simulink model "Half_car_model_susp_bump_tyre"  (R2025b)
settings: Solver=VariableStepAuto  StartTime=0.0  StopTime=15  RelTol=1e-3
values from neighbouring files (symbols this model uses):
  A_N = double(vpa(subs(A_0, symbol_vars , numeric_vals), 6))    [half_car_active_suspensions_bump.m]
  B1_N = double(vpa(subs(B1_0, symbol_vars , numeric_vals), 6))    [half_car_active_suspensions_bump.m]
  B2_N = double(vpa(subs(B2_0, symbol_vars , numeric_vals), 6))    [half_car_active_suspensions_bump.m]
  bump_t_dist = (df+dr)/1    (= 3)    [half_car_active_suspensions_bump.m]
  C_N = double(vpa(subs(C_0, symbol_vars , numeric_vals), 6))    [half_car_active_suspensions_bump.m]
  CE_N = double(vpa(subs(CE_0, symbol_vars , numeric_vals), 6))    [half_car_active_suspensions_bump.m]
  D1_N = double(vpa(subs(D1_0, symbol_vars , numeric_vals), 6))    [half_car_active_suspensions_bump.m]
  D2_N = double(vpa(subs(D2_0, symbol_vars , numeric_vals), 6))    [half_car_active_suspensions_bump.m]
  DE2_N = double(vpa(subs(DE2_0, symbol_vars , numeric_vals), 6))    [half_car_active_suspensions_bump.m]
  Delta0 = -(m)*g/(2*k)    (= -0.17658)    [half_car_active_suspensions_bump.m]
  Delta0_W = -(m+mwf*2)*g/(2*ktf)    (= -0.0230535)    [half_car_active_suspensions_bump.m]
  Ko = place(A_N', C_N', poles_obs)'    [half_car_active_suspensions_bump.m]
  Ks = [Ks_c, zeros(2, 4)]    [half_car_active_suspensions_bump.m]
  Ks_obs = lqr(A_stabile, B1_N, Q, R)    [half_car_active_suspensions_bump.m]
  par_numeric = [ m, k, beta, ell0, g, df, dr, J, mwf, mwr, ktf, ktr ]    [half_car_active_suspensions_bump.m]
  u0 = [0; 0]    [half_car_active_suspensions_bump.m]
  x0 = [  Delta0 + Delta0_W ... (first row only)    [half_car_active_suspensions_bump.m]
  x0_lin = [ ... (first row only)    [half_car_active_suspensions_bump.m]
libraries: simulink x1
settings Model: LastModifiedBy=alex2

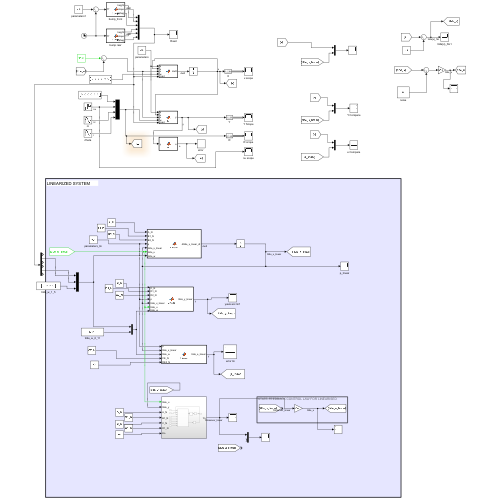
[thumbnail: Simulink's stored preview of the top-level diagram]
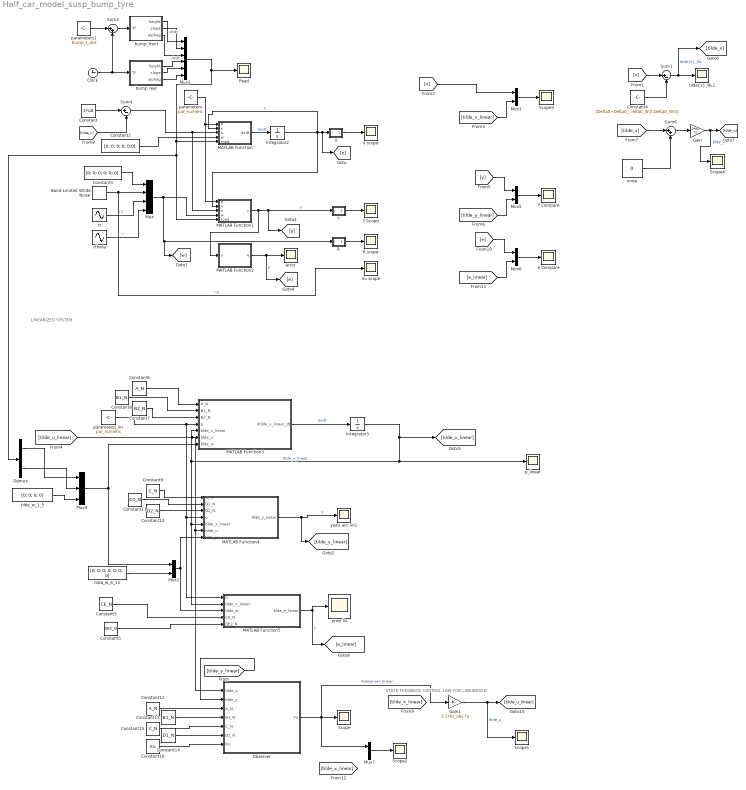
== system Half_car_model_susp_bump_tyre ==
  note: STATE-FEEDBACK CONTROL LAW FOR LINEARISED
  note: LINEARIZED SYSTEM
  " error lin" : Scope
      settings: ActiveDisplayYMinimum=-1  ActiveDisplayYMaximum=1  DataLoggingVariableName=ScopeData8
  Band-Limited White Noise : simulink/Sources/Band-Limited White Noise  Cov="1*[0.00001*1e-2; 0.00001*1e-2;  0.00001*1e-2; 0.00001*1e-2; 0.00001*1e-2]"  Ts=1e-2  seed=[23341; 31826; 11111; 81818; 00001]
  Clock : Clock
  Constant : Constant  Value=1*u0
  Constant1 : Constant  Value=[0; 0; 0; 0; 0; 0]
  Constant10 : Constant  Value=D2_N
  Constant11 : Constant  Value=D1_N
  Constant12 : Constant  Value=A_N
  Constant13 : Constant  Value=B1_N
  Constant14 : Constant  Value=D1_N
  Constant15 : Constant  Value=C_N
  Constant16 : Constant  Value=Ko
  Constant2 : Constant  Value=[0; 0; 0; 0; 0;0]
  Constant3 : Constant  Value=CE_N
  Constant4 : Constant  Value=[Delta0+Delta0_W;0;0;0;Delta0_W;0;Delta0_W;0]
  Constant5 : Constant  Value=DE2_N
  Constant6 : Constant  Value=A_N
  Constant7 : Constant  Value=B2_N
  Constant8 : Constant  Value=B1_N
  Constant9 : Constant  Value=C_N
  Demux : Demux  Outputs=6
  Gain : Gain  Gain=0*Ks  Multiplication=Matrix(K*u)
  Gain1 : Gain  Gain=3.5*Ks_obs  Multiplication=Matrix(K*u)
  Integrator2 : Integrator  InitialCondition=x0
  Integrator3 : Integrator  InitialCondition=x0_lin
  MATLAB Function : MATLAB Function  TreatAsAtomicUnit=on
  MATLAB Function1 : MATLAB Function  TreatAsAtomicUnit=on
  MATLAB Function2 : MATLAB Function  TreatAsAtomicUnit=on
  MATLAB Function3 : MATLAB Function  TreatAsAtomicUnit=on
  MATLAB Function4 : MATLAB Function  TreatAsAtomicUnit=on
  MATLAB Function5 : MATLAB Function  TreatAsAtomicUnit=on
  Mux : Mux
  Mux{1..2,5..7} (5 alike) : Mux  Inputs=2
  Mux3 : Mux  Inputs=6
  Mux4 : Mux  Inputs=3
  Observer : Subsystem
  R : Subsystem
  R scope : Scope
      settings: ActiveDisplayYMinimum=-1  ActiveDisplayYMaximum=1  DataLoggingVariableName=ScopeData5
  Road : Scope
      settings: ActiveDisplayYMinimum=-0.19634954084936207  ActiveDisplayYMaximum=0.19634954084936207
  Scope{,1..4} (5 alike) : Scope
      Scope settings: ActiveDisplayYMinimum=-1  ActiveDisplayYMaximum=1  DataLoggingVariableName=ScopeData13
      Scope1 settings: ActiveDisplayYMinimum=-1  ActiveDisplayYMaximum=1  DataLoggingVariableName=ScopeData14
      Scope2 settings: ActiveDisplayYMinimum=-1.3124834996188637  ActiveDisplayYMaximum=1.3703591925048633  DataLoggingVariableName=ScopeData15
      Scope3 settings: ActiveDisplayYMinimum=-0.26211296691734631  ActiveDisplayYMaximum=0.090134709396633
      Scope4 settings: ActiveDisplayYMinimum=-1  ActiveDisplayYMaximum=1  DataLoggingVariableName=ScopeData16
  Sum1 : Sum  Inputs=|+-
  Sum2 : Sum  Inputs=|++
  Sum4 : Sum  Inputs=|+-
  Sum6 : Sum  Inputs=|++
  X : Subsystem
  Y : Subsystem
  Y Compare : Scope
      settings: ActiveDisplayYMinimum=-9.06978679583773  ActiveDisplayYMaximum=22.15478865739642  DataLoggingVariableName=ScopeData11
  Y Scope : Scope
      settings: ActiveDisplayYMinimum=-1  ActiveDisplayYMaximum=1  DataLoggingVariableName=ScopeData3
  bump rear : MATLAB Function  TreatAsAtomicUnit=on
  bump_front : MATLAB Function  TreatAsAtomicUnit=on
  e Compare : Scope
      settings: ActiveDisplayYMinimum=-0.3208309292462625  ActiveDisplayYMaximum=0.34771769859425983  DataLoggingVariableName=ScopeData12
  "error " : Scope
      settings: ActiveDisplayYMinimum=-1  ActiveDisplayYMaximum=1  DataLoggingVariableName=ScopeData6
  noise : Constant  Value=0
  nu scope : Scope
      settings: DataLoggingVariableName=ScopeData7
  p_linear : Scope
      settings: ActiveDisplayYMinimum=-0.03749851288711617  ActiveDisplayYMaximum=0.066646245320476569  DataLoggingVariableName=ScopeData9
  parameters : Constant  Value=par_numeric  VectorParams1D=off
  parameters1 : Constant  Value=bump_t_dist  VectorParams1D=off
  parameters_lin : Constant  Value=par_numeric
  rtheta : Sin  Amplitude=0  Frequency=0  SampleTime=0
  rz : Sin  Amplitude=0  Frequency=0  SampleTime=0
  tilde_w_1_5 : Constant  Value=[0; 0; 0; 0]
  tilde_w_6_11 : Constant  Value=[0; 0; 0; 0; 0; 0; 0]
  "tilde{x}_NL1" : Scope
      settings: ActiveDisplayYMinimum=-4.93552  ActiveDisplayYMaximum=2.55492  DataLoggingVariableName=ScopeData4
  x scope : Scope
      settings: ActiveDisplayYMinimum=-0.66741875872169254  ActiveDisplayYMaximum=0.73384060742897  DataLoggingVariableName=ScopeData2
  yaxis acc lin1 : Scope
      settings: ActiveDisplayYMinimum=-1  ActiveDisplayYMaximum=1  DataLoggingVariableName=ScopeData10
  wires:
  Clock/1 -> Sum2/2, bump rear/1(Tf)
  bump_front/2(slope) -> Mux3/2
  Sum2/1 -> bump_front/1(Tf)
  parameters1/1 -> Sum2/1
  Mux3/1 -> Road/1, MATLAB Function/5(road), Demux/1, MATLAB Function1/5(road)
  bump_front/1(height) -> Mux3/1  "dxdt"
  Constant/1 -> Sum4/1
  Sum4/1 -> MATLAB Function1/3(u), MATLAB Function/3(u)
  Constant2/1 -> MATLAB Function/4(w)
  MATLAB Function/1(dxdt) -> Integrator2/1  "dxdt"
  MATLAB Function1/1(y) -> Y/1(i), [y], MATLAB Function2/1(y)  "y"
  Constant1/1 -> Mux/1
  rtheta/1 -> Mux/4  "r"
  parameters/1 -> MATLAB Function1/1(p), MATLAB Function/1(p)
  Band-Limited White Noise/1 -> nu scope/1, Mux/2  "nu"
  rz/1 -> Mux/3  "rz"
  Mux/1 -> [w], R/1(i), MATLAB Function1/4(w)
  MATLAB Function2/1(e) -> [e], "error "/1  "e"
  Sum6/1 -> Gain/1
  [tilde_x] -> Sum6/1
  [x] -> Sum1/1
  Constant4/1 -> Sum1/2
  Sum1/1 -> [tilde_x], "tilde{x}_NL1"/1  "tilde{x}_NL"
  noise/1 -> Sum6/2
  [tilde_x_linear] -> Mux1/2
  Gain/1 -> Scope4/1, [tilde_u]  "tilde_u"
  Mux1/1 -> Scope3/1
  [tilde_u] -> Sum4/2
  Integrator2/1 -> [x], X/1(i), MATLAB Function1/2(x), MATLAB Function/2(x)  "x"
  X/1(o) -> x scope/1
  Y/1(o) -> Y Scope/1
  R/1(o) -> R scope/1
  tilde_w_6_11/1 -> Mux2/2
  parameters_lin/1 -> MATLAB Function3/4(p), MATLAB Function5/1(p), MATLAB Function4/4(p)
  [tilde_u_linear] -> Observer/1(tilde_u), MATLAB Function4/6(tilde_u), MATLAB Function3/6(tilde_u)
  Gain1/1 -> Scope1/1, [tilde_u_linear]  "tilde_u"
  MATLAB Function4/1(tilde_y_linear) -> [tilde_y_linear], yaxis acc lin1/1  "y"
  Mux2/1 -> MATLAB Function4/7(tilde_w), MATLAB Function5/3(tilde_w)
  MATLAB Function5/1(tilde_e_linear) -> " error lin"/1, [e_linear]  "y"
  Constant3/1 -> MATLAB Function5/4(CE_N)
  Constant5/1 -> MATLAB Function5/5(DE2_N)
  Constant7/1 -> MATLAB Function3/3(B2_N)
  Constant6/1 -> MATLAB Function3/1(A_N)
  Constant8/1 -> MATLAB Function3/2(B1_N)
  Constant10/1 -> MATLAB Function4/3(D2_N)
  Constant11/1 -> MATLAB Function4/2(D1_N)
  Constant9/1 -> MATLAB Function4/1(C_N)
  Mux4/1 -> MATLAB Function3/7(tilde_w), Mux2/1
  tilde_w_1_5/1 -> Mux4/3
  Demux/2 -> Mux4/1
  bump_front/3(alphag) -> Mux3/3
  bump rear/1(height) -> Mux3/4  "dxdt"
  bump rear/2(slope) -> Mux3/5
  bump rear/3(alphag) -> Mux3/6
  Demux/5 -> Mux4/2
  MATLAB Function3/1(dtilde_x_linear_dt) -> Integrator3/1  "dxdt"
  Integrator3/1 -> p_linear/1, MATLAB Function3/5(tilde_x_linear), MATLAB Function5/2(tilde_x_linear), MATLAB Function4/5(tilde_x_linear), [tilde_x_linear]  "tilde_x_linear"
  [y] -> Mux5/1
  Mux5/1 -> Y Compare/1
  [tilde_y_linear] -> Mux5/2
  Mux6/1 -> e Compare/1
  [e] -> Mux6/1
  [e_linear] -> Mux6/2
  [tilde_y_linear] -> Observer/2(tilde_y)
  Observer/1(Yo) -> Mux7/1, Gain1/1, Scope/1  "Yobserver_linear"
  Constant16/1 -> Observer/7(Ko)
  Constant14/1 -> Observer/6(D1_N)
  Constant15/1 -> Observer/5(C_N)
  Constant13/1 -> Observer/4(B1_N)
  Constant12/1 -> Observer/3(A_N)
  Mux7/1 -> Scope2/1
  [x] -> Mux1/1

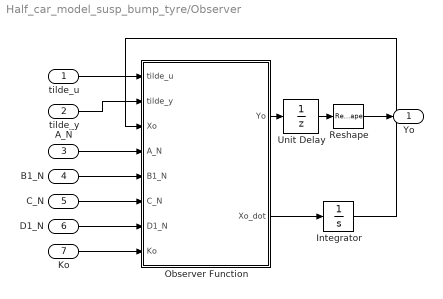
== system Half_car_model_susp_bump_tyre/Observer ==
  tilde_u : Inport
  tilde_y : Inport  Port=2
  A_N : Inport  Port=3
  B1_N : Inport  Port=4
  C_N : Inport  Port=5
  D1_N : Inport  Port=6
  Ko : Inport  Port=7
  Integrator : Integrator  InitialCondition=x0_lin
  Observer Function : MATLAB Function  TreatAsAtomicUnit=on
  Reshape : Reshape  OutputDimensionality=Customize  OutputDimensions=[12]
  Unit Delay : UnitDelay  SampleTime=0.01  HasFrameUpgradeWarning=on
  Yo : Outport
  wires:
  Observer Function/2(Xo_dot) -> Integrator/1
  Integrator/1 -> Observer Function/3(Xo)
  tilde_u/1 -> Observer Function/1(tilde_u)
  tilde_y/1 -> Observer Function/2(tilde_y)
  A_N/1 -> Observer Function/4(A_N)
  B1_N/1 -> Observer Function/5(B1_N)
  C_N/1 -> Observer Function/6(C_N)
  D1_N/1 -> Observer Function/7(D1_N)
  Ko/1 -> Observer Function/8(Ko)
  Reshape/1 -> Yo/1
  Observer Function/1(Yo) -> Unit Delay/1
  Unit Delay/1 -> Reshape/1

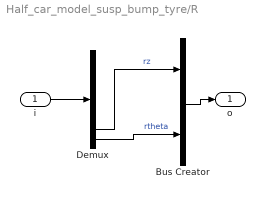
== system Half_car_model_susp_bump_tyre/R ==
  i : Inport
  Bus Creator : BusCreator  Inputs=2
  Demux : Demux  Outputs=9
  o : Outport
  wires:
  i/1 -> Demux/1
  Bus Creator/1 -> o/1
  Demux/9 -> Bus Creator/2  "rtheta"
  Demux/8 -> Bus Creator/1  "rz"

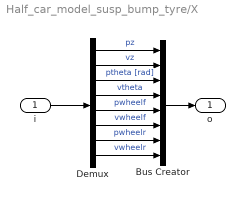
== system Half_car_model_susp_bump_tyre/X ==
  i : Inport
  Bus Creator : BusCreator  Inputs=8
  Demux : Demux  Outputs=8
  o : Outport
  wires:
  Demux/8 -> Bus Creator/8  "vwheelr"
  Demux/4 -> Bus Creator/4  "vtheta"
  Demux/1 -> Bus Creator/1  "pz"
  Demux/2 -> Bus Creator/2  "vz"
  Demux/5 -> Bus Creator/5  "pwheelf"
  Demux/3 -> Bus Creator/3  "ptheta [rad]"
  Demux/7 -> Bus Creator/7  "pwheelr"
  Demux/6 -> Bus Creator/6  "vwheelf"
  i/1 -> Demux/1
  Bus Creator/1 -> o/1

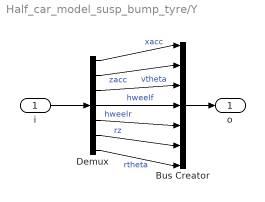
== system Half_car_model_susp_bump_tyre/Y ==
  i : Inport
  Bus Creator : BusCreator  Inputs=7
  Demux : Demux  Outputs=7
  o : Outport
  wires:
  Demux/4 -> Bus Creator/4  "hweelf"
  Demux/1 -> Bus Creator/1  "xacc"
  Demux/2 -> Bus Creator/2  "zacc"
  Demux/3 -> Bus Creator/3  "vtheta"
  i/1 -> Demux/1
  Bus Creator/1 -> o/1
  Demux/7 -> Bus Creator/7  "rtheta"
  Demux/6 -> Bus Creator/6  "rz"
  Demux/5 -> Bus Creator/5  "hweelr"

== matlab function Half_car_model_susp_bump_tyre/MATLAB Function1 ==
  data: p input; x input; u input; y output; w input; road input
function y = h(p,x, u, w, road)

%% parameters
m = p(1);      % [kg] mass
k = p(2);    % [N/m] spring stiffness
beta = p(3);   % [N/(m/s)] damper coeff.
ell0 = p(4);   % [m] 0-load lenght
g = p(5);   % [m/s^2] gravity acceleration
df = p(6);     % [m] distance between center of mass and front
dr = p(7);     % [m] distance between center of mass and rear
J = p(8);      % [kg*m^2] Moment of interti
mwf = p(9);     %[kg] massa ruote AV (asse completo)
mwr = p(10);    %[kg] massa ruote AP (asse completo)
ktf = p(11);   %[N/m] rigidezza pneumatici AV (asse)
ktr = p(12);  %[N/m] rigidezza pneumatici AP (asse)

%% state
pz = x(1);        % [m] heigth of the center of mass of the car 
vz = x(2);        % [m/s] speed of the center of mass of the car 
ptheta = x(3);    % [Rad] pitch angle of the car 
vtheta = x(4);    % [Rad/s] angular speed of the car 
hwheelf = x(5);
dhwheelf = x(6);
hwheelr = x(7);
dhwheelr = x(8);


zroad_f = road(1);
thetaroad_f = road(2);
alphag_f = road(3);

zroad_r = road(4);    
thetaroad_r = road(5); 
alphag_r = w(6);

%% disturbance
zroad_f_dot = w(1);
zroad_r_dot = w(2);
% alphag_f = w(3);
% alphag_r = w(4);
fwfront = w(5);
fwrear = w(6);

%todo: Vedere se servono due disturbi 

%% state evolution
 
s1 = (pz-hwheelf)+df*(sin(ptheta)-sin(thetaroad_f)); % height of front suspension
s3 = (pz-hwheelr)-dr*(sin(ptheta)-sin(thetaroad_r)); % height of rear suspension

% s2 = (vz-dhwheelf)+df*(vtheta*cos(ptheta)-thetaroad_f*cos(thetaroad_f)); % height speed of front suspension
% s4 = (vz-dhwheelr)-dr*(vtheta*cos(ptheta)-thetaroad_r*cos(thetaroad_r)); % height speed of rear suspension

s2 = (vz-dhwheelf)+df*(vtheta*cos(ptheta)-alphag_f*cos(thetaroad_f)); % height speed of front suspension
s4 = (vz-dhwheelr)-dr*(vtheta*cos(ptheta)-alphag_r*cos(thetaroad_r)); % height speed of rear suspension

lf = s1 + ell0;
lr = s3 + ell0;

%% Forze sospensioni & pneumatici
fsf = -k*s1 - beta*s2;      % sospensione anteriore
fsr = -k*s3 - beta*s4;      % sospensione posteriore

ftf =  ktf*(zroad_f - hwheelf); % pneumatico anteriore (no damping)
ftr =  ktr*(zroad_r - hwheelr); % pneumatico posteriore (no damping)

fmgf = - mwf * g;
fmgr = - mwf * g;

%% Ripartizione attuatori u1,u2 -> forze su body alle estremità
% [faf + far = u1;   df*faf - dr*far = u2]
faf = (u(2) + dr*u(1))/(df + dr);      % forza attuatore anteriore
far = (df*u(1) - u(2))/(df + dr);      % forza attuatore posteriore

%% Dinamica: corpo
f2 = -g + (fsf + fsr + u(1))/m;                                     % acc. verticale
f4 = (df*fsf - dr*fsr + u(2) + fwfront*lf + fwrear*lr)/J;           % pitch

%% Dinamica: ruote (masse non sospese)
% segno: su ruota, verso +z è (forza pneumatico - forza sospensione - attuatore locale)
f_wf = (ftf - fsf - faf + fmgf)/mwf;   % acc. ruota ant
f_wr = (ftr - fsr - far + fmgr)/mwr;   % acc. ruota post


nuy = w(7);
nuz = w(7);
nug = w(7);
nuf = w(7);
nur = w(7);

%% reference
rz = w(8);
rtheta=w(9);


%% output
y = [sin(x(3))*(f2 + g) + cos(x(3)) * ((fwrear + fwfront) / m)+nuy; % h_xacc
     cos(x(3))*(f2 + g) - sin(x(3)) * ((fwrear + fwfront) / m)+nuz; % h_zacc  se facciamo cosi ci da in condizioni stazionarie Zaxisacc=9.81, se vogliamo il valore negativo mettere "-" davanti a coseno 
     x(4)+nug;                                                      % h_vtheta
     s1+nuf;                                                        % h_hweelf
     s3+nur;                                                        % h_hweelf
     rz;                                                            % h_rz
     rtheta];                                                       % h_rtheta
end

== matlab function Half_car_model_susp_bump_tyre/MATLAB Function ==
  data: p input; x input; u input; dxdt output; w input; road input
function dxdt = f(p,x,u,w,road)

%% parameters
m = p(1);      % [kg] mass
k = p(2);    % [N/m] spring stiffness
beta = p(3);   % [N/(m/s)] damper coeff.
ell0 = p(4);   % [m] 0-load lenght
g = p(5);   % [m/s^2] gravity acceleration
df = p(6);     % [m] distance between center of mass and front
dr = p(7);     % [m] distance between center of mass and rear
J = p(8);      % [kg*m^2] Moment of interti
mwf = p(9);     %[kg] massa ruote AV (asse completo)
mwr = p(10);    %[kg] massa ruote AP (asse completo)
ktf = p(11);   %[N/m] rigidezza pneumatici AV (asse)
ktr = p(12);  %[N/m] rigidezza pneumatici AP (asse)

%% state
pz = x(1);        % [m] heigth of the center of mass of the car 
vz = x(2);        % [m/s] speed of the center of mass of the car 
ptheta = x(3);    % [Rad] pitch angle of the car 
vtheta = x(4);    % [Rad/s] angular speed of the car 
hwheelf = x(5);
dhwheelf = x(6);
hwheelr = x(7);
dhwheelr = x(8);


zroad_f = road(1);


zroad_r = road(4);    
thetaroad_r = 0;
thetaroad_f = 0;


%% disturbance
zroad_f_dot = w(1);
zroad_r_dot = w(2);
% alphag_f = w(3);
% alphag_r = w(4);
fwfront = w(5);
fwrear = w(6);

%todo: Vedere se servono due disturbi 

%% state evolution
 
s1 = (pz-hwheelf)+df*(sin(ptheta)-sin(thetaroad_f)); % height of front suspension
s3 = (pz-hwheelr)-dr*(sin(ptheta)+sin(thetaroad_r)); % height of rear suspension

% s2 = (vz-dhwheelf)+df*(vtheta*cos(ptheta)-thetaroad_f*cos(thetaroad_f)); % height speed of front suspension
% s4 = (vz-dhwheelr)-dr*(vtheta*cos(ptheta)-thetaroad_r*-cos(thetaroad_r)); % height speed of rear suspension

s2 = (vz - dhwheelf) + df * vtheta;
s4 = (vz - dhwheelr) - dr * vtheta;

lf = s1 + ell0;
lr = s3 + ell0;

%% Forze sospensioni & pneumatici
fsf = -k*s1 - beta*s2;      % sospensione anteriore
fsr = -k*s3 - beta*s4;      % sospensione posteriore

ftf =  ktf*(zroad_f - hwheelf); % pneumatico anteriore (no damping)
ftr =  ktr*(zroad_r - hwheelr); % pneumatico posteriore (no damping)

fmgf = - mwf * g;
fmgr = - mwf * g;

%% Ripartizione attuatori u1,u2 -> forze su body alle estremità
% [faf + far = u1;   df*faf - dr*far = u2]
faf = (u(2) + dr*u(1))/(df + dr);      % forza attuatore anteriore
far = (df*u(1) - u(2))/(df + dr);      % forza attuatore posteriore

%% Dinamica: corpo
f2 = -g + (fsf + fsr + faf + far)/m;                  %acc vertt
f4 = (df*(fsf + faf) - dr*(fsr + far))/J;;           % pitch

%% Dinamica: ruote (masse non sospese)
% segno: su ruota, verso +z è (forza pneumatico - forza sospensione - attuatore locale)
f_wf = (ftf - fsf - faf + fmgf)/mwf;   % acc. ruota ant
f_wr = (ftr - fsr - far + fmgr)/mwr;   % acc. ruota post


%f2 = -g + (((-k*(s1-ell0)-beta*s2)+(-k*(s3-ell0)-beta*s4))+u(1))/m; %  con  ell0
%f4 = (df*(-k*(s1-ell0)-beta*s2)-dr*(-k*(s3-ell0)-beta*s4)+u(2)+fwfront*lf+fwrear*lr)/J; %


%f2 = -g + (((-k*(s1)-beta*s2)+(-k*(s3)-beta*s4))+u(1))/m; %  senza ell0
%f4 = (df*(-k*(s1)-beta*s2)-dr*(-k*(s3)-beta*s4)+u(2)+fwfront*lf+fwrear*lr)/J; %

% dxdt = [vz;
%         f2-zgsecond; 
%         x(4);
%         f4;
%         x(6);
%         alphag];
        
dxdt = [ ...
    vz;                   % pz_dot
    f2;                   % vz_dot
    vtheta;               % ptheta_dot
    f4;                   % vtheta_dot
    dhwheelf;             % zwf_dot
    f_wf;                 % vwf_dot
    dhwheelr;             % zwr_dot
    f_wr ]                % vwr_dot




end

== matlab function Half_car_model_susp_bump_tyre/MATLAB Function2 ==
  data: y input; e output
function e = E(y)

df = 1;     % [m] distance between center of mass and front
dr = 1;     % [m] distance between center of mass and rear


yy = y(1); % output of h block yaxisacc 
yz = y(2); % output of h block zaxisacc 
yg = y(3); % output of h block gyro
yf = y(4); % output of h block pot. front
yr = y(5); % output of h block pot. rear
 
%% ref
rz = y(6);
rtheta = y(7);

e = [
    (yf*dr+yr*df)/(dr+df)-rz; 
    asin((yy)/(sqrt(yy^2+yz^2)))-rtheta];
end

== matlab function Half_car_model_susp_bump_tyre/MATLAB Function3 ==
  data: A_N input; B1_N input; B2_N input; p input; tilde_x_linear input; tilde_u input; dtilde_x_linear_dt output; tilde_w input
function dtilde_x_linear_dt = Linear(A_N, B1_N, B2_N, p,tilde_x_linear,tilde_u,tilde_w)

dtilde_x_linear_dt = A_N*tilde_x_linear+B1_N*tilde_u+B2_N*tilde_w;
end

== matlab function Half_car_model_susp_bump_tyre/MATLAB Function4 ==
  data: C_N input; D1_N input; D2_N input; p input; tilde_x_linear input; tilde_u input; tilde_y_linear output; tilde_w input
function tilde_y_linear = Linear(C_N, D1_N, D2_N, p,tilde_x_linear,tilde_u,tilde_w)

% 
% %% parameters
% m = p(1);      % [kg] mass
% k = p(2);    % [N/m] spring stiffness
% beta = p(3);   % [N/(m/s)] damper coeff.
% ell0 = p(4);   % [m] 0-load lenght
% g = p(5);   % [m/s^2] gravity acceleration
% df = p(6);     % [m] distance between center of mass and front
% dr = p(7);     % [m] distance between center of mass and rear
% J = p(8);      % [kg*m^2] Moment of interti
% 
% 
% 
% C = [0, 0, g, 0, 0, 0;
%     -2*k/m, -2*beta/m, -k*(df-dr)/m, -beta*(df-dr)/m, k*(df-dr)/m, beta*(df-dr)/m;
%     0, 0, 0, 1, 0, 0;
%     1, 0, df, 0, -df, 0;
%     1, 0, -dr, 0, dr, 0];
% 
% 
% D1 = [0,0;
%      1/m, 0;
%      0,0;
%      0,0;
%      0,0];
% 
% D2 = [0,0,1/m,1/m,1,0,0,0,0,0,0;
%       0,0,0,0,0,1,0,0,0,0,0;
%       0,0,0,0,0,0,1,0,0,0,0;
%       0,0,0,0,0,0,0,1,0,0,0;
%       0,0,0,0,0,0,0,0,1,0,0];

%% state evolution
% tilde_y_linear = C*tilde_x_linear+D1*tilde_u+D2*tilde_w;

tilde_y_linear = C_N*tilde_x_linear+D1_N*tilde_u+D2_N*tilde_w;
end

== matlab function Half_car_model_susp_bump_tyre/MATLAB Function5 ==
  data: p input; tilde_x_linear input; tilde_e_linear output; tilde_w input; CE_N input; DE2_N input
function tilde_e_linear = Linear(p,tilde_x_linear,tilde_w, CE_N, DE2_N)

% 
% %% parameters
% m = p(1);      % [kg] mass
% k = p(2);    % [N/m] spring stiffness
% beta = p(3);   % [N/(m/s)] damper coeff.
% ell0 = p(4);   % [m] 0-load lenght
% g = p(5);   % [m/s^2] gravity acceleration
% df = p(6);     % [m] distance between center of mass and front
% dr = p(7);     % [m] distance between center of mass and rear
% J = p(8);      % [kg*m^2] Moment of interti
% 
% 
% 
% Ce = [1,0,0,0,0,0;
%       0,0,1,0,0,0];
% 
% 
% 
% De2 = [0,0,0,0,0,0,0,dr/(dr+df),df/(dr+df),-1,0;
%        0,0, 1/(m*g),1/(m*g),1/g,0,0,0,0,0,-1];


%% state evolution
% tilde_e_linear = Ce*tilde_x_linear+De2*tilde_w;

tilde_e_linear = CE_N*tilde_x_linear+DE2_N*tilde_w;
end

== matlab function Half_car_model_susp_bump_tyre/bump rear ==
  data: height output; slope output; Tf input; alphag output
function [height, slope, alphag] = bump(Tf)
    % Parametri
    a = 0.10;       % Ampiezza del bump (m)
    V = 10;         % Velocità del veicolo (m/s)
    lambda = 10;     % Lunghezza dell'onda del bump (m)
    % Tspan = 5;    % Durata della simulazione (s) - Parametro non usato in questa funzione
    T1 = 10;        % Tempo di inizio del bump (s)
    T2 = T1 + lambda/V; % Tempo di fine del bump (s)

    % Controllo manuale per definire l'intervallo del bump
    is_on_bump = (Tf >= T1) & (Tf <= T2);
    
    % Termine comune A = (2*pi*V)/lambda
    A = (2*pi*V)/lambda;
    
    % Termine comune B = (2*pi*V*Tf)/lambda
    B = A * Tf;

    % Calcola l'altezza della strada (height)
    height = (a/2) * (1 - cos(B)) .* is_on_bump; 
    
    % Calcola la pendenza della strada (slope - derivata prima)
    % slope = (a/2) * A * sin(B)
    slope = (a/2) * A .* sin(B) .* is_on_bump; 

    % Calcola la derivata della pendenza (derivata_slope - derivata seconda)
    % derivata_slope = (a/2) * A^2 * cos(B)
    alphag = (a/2) * (A^2) .* cos(B) .* is_on_bump; 
end



% function [height, slope] = continuous_45deg_slope(Tf)
%     % --- Parametro ---
%     V = 20;         % Velocità del veicolo (m/s)
%     m = -1;         % Pendenza fisica della strada (-45 gradi)
% 
%     % --- Calcolo della Pendenza (Slope) ---
%     % La pendenza rispetto al tempo (d(height)/dTf) è costante.
%     slope = m * V; 
% 
%     % --- Calcolo dell'Elevazione (Height) ---
%     % L'altezza è l'integrale della pendenza rispetto al tempo (assumendo height=0 per Tf=0).
%     % height(Tf) = integral(slope * dTf) = (m * V) * Tf
%     height = (m * V) * Tf; 
% end

== matlab function Half_car_model_susp_bump_tyre/bump_front ==
  data: height output; slope output; Tf input; alphag output
function [height, slope, alphag] = bump(Tf)
    % Parametri
    a = 0.10;       % Ampiezza del bump (m)
    V = 10;         % Velocità del veicolo (m/s)
    lambda = 10;     % Lunghezza dell'onda del bump (m)
    % Tspan = 5;    % Durata della simulazione (s) - Parametro non usato in questa funzione
    T1 = 5;        % Tempo di inizio del bump (s)
    T2 = T1 + lambda/V; % Tempo di fine del bump (s)

    % Controllo manuale per definire l'intervallo del bump
    is_on_bump = (Tf >= T1) & (Tf <= T2);
    
    % Termine comune A = (2*pi*V)/lambda
    A = (2*pi*V)/lambda;
    
    % Termine comune B = (2*pi*V*Tf)/lambda
    B = A * Tf;

    % Calcola l'altezza della strada (height)
    height = (a/2) * (1 - cos(B)) .* is_on_bump; 
    
    % Calcola la pendenza della strada (slope - derivata prima)
    % slope = (a/2) * A * sin(B)
    slope = (a/2) * A .* sin(B) .* is_on_bump; 

    % Calcola la derivata della pendenza (derivata_slope - derivata seconda)
    % derivata_slope = (a/2) * A^2 * cos(B)
    alphag = (a/2) * (A^2) .* cos(B) .* is_on_bump; 
end


% function [height, slope] = continuous_45deg_slope(Tf)
%     % --- Parametro ---
%     V = 20;         % Velocità del veicolo (m/s)
%     m = -1;         % Pendenza fisica della strada (-45 gradi)
% 
%     % --- Calcolo della Pendenza (Slope) ---
%     % La pendenza rispetto al tempo (d(height)/dTf) è costante.
%     slope = m * V; 
% 
%     % --- Calcolo dell'Elevazione (Height) ---
%     % L'altezza è l'integrale della pendenza rispetto al tempo (assumendo height=0 per Tf=0).
%     % height(Tf) = integral(slope * dTf) = (m * V) * Tf
%     height = (m * V) * Tf; 
% end

== matlab function Half_car_model_susp_bump_tyre/Observer/Observer Function ==
  data: tilde_u input; tilde_y input; Yo output; Xo_dot output; Xo input; A_N input; B1_N input; C_N input; D1_N input; Ko input
function [Yo, Xo_dot] = fcn(tilde_u, tilde_y, Xo, A_N, B1_N, C_N, D1_N, Ko)
    % tilde_u: Ingressi di controllo [2x1] (u1, u2)
    % tilde_y: Misure dai sensori [5x1] (ax, az, vtheta, s1, s3)
    % Xo:      Stato stimato attuale [12x1]
    % Ko:      Guadagno dell'osservatore [12x5]
    
    %% 1. Calcolo dell'uscita stimata (Cosa l'osservatore "pensa" di leggere)
    % y_hat = C * x_stimato + D * u
    tilde_y_hat = C_N * Xo + D1_N * tilde_u;
    
    %% 2. Calcolo dell'errore di stima (Residuo)
    % Differenza tra misura reale del sensore e misura prevista dal modello
    e_y = tilde_y - tilde_y_hat;
    
    %% 3. Dinamica dell'Observer (Equazione di Luenberger)
    % Xo_dot = A*Xo + B*u + Ko*(y - y_hat)
    % Il termine Ko * e_y è quello che corregge lo stato verso la realtà
    Xo_dot = A_N * Xo + B1_N * tilde_u + Ko * e_y;
    
    %% 4. Uscita dell'Observer
    % In questo caso Yo è lo stato stimato completo che va allo stabilizzatore
    % Non serve reshape se Xo è già un vettore colonna 12x1
    Yo = Xo; 
    
end
